simulink model "acados_test_old"  (R2017b)
settings: Solver=FixedStepDiscrete  StartTime=0.0  StopTime=200  FixedStep=1  RelTol=1e-3
PostLoadFcn:
  | , if any(exist('dsrtsu_mdlpostloadfcn', 'file') == [2, 3, 6]), try dsrtsu_mdlpostloadfcn('Execute', bdroot); catch fprintf('Error in PostLoadFcn (dsrtsu_mdlpostloadfcn) for model "%s":\n %s\n', bdroot, lasterr); end, end,
Description:
  | Standard RTI1401 template.
  | Supported MATLAB version:  R2017b.
settings Model: Tag=RTI1401  DSRTSU_INTERNAL_RTI_VER=520  DSRTSU_INTERNAL_RTI_TYPE=rti1401  RTICANMMDATA=struct('GeneralSetupData',struct('modelroot','D:\dSpace_Acados_Test','generalsettings',struct('filesettings',struct('destfolder',struct('Name','RTICANMM_FILES','Check',1),'buildfolder',struct('Name','.','Check',1),'AbsDestfolder',struct('Name','D:\dSpace_Acados_Test\RTICANMM_FILES'),'AbsBuildfolder',struct('Name','D:\dSpace_Acados_Test'))),'options',struct('addpaths',1,'rmpaths',1,'addtrcexclusion',logical(1),'cannavigator',struct('checkmonitoring',0),'show_usrtrc',0,'use_usrtrc',0),'advanced',struct('options',ones(1,100)),'MPSetup',{{}},'RTI',struct('Type','RTI1401','Ver','7.10','Date','02-May-2018'),'modelname','acados_test','block','acados_test'))  DSRTSU_INTERNAL_RTIFPGA=110  Creator=fleqscar  LastModifiedBy=fleqscar
settings SolverCC: AlgebraicLoopSolver=LineSearch
settings OptimizationCC: BlockReduction=off  OptimizeBlockIOStorage=off  BufferReuse=off  GlobalBufferReuse=off  ExpressionFolding=off  LocalBlockOutputs=off
settings HardwareCC: ProdBitPerPointer=32  ProdBitPerSizeT=32  ProdBitPerPtrDiffT=32  ProdLargestAtomicInteger=Integer  ProdEndianess=BigEndian  ProdWordSize=32  ProdHWDeviceType=Custom Processor->Custom  TargetIntDivRoundTo=Zero  TargetEndianess=BigEndian  TargetHWDeviceType=Custom Processor->Custom
settings SFSimCC: MATLABDynamicMemAlloc=off
settings RTWCC: SystemTargetFile=rti1401.tlc  MakeCommand=make_rti  TemplateMakefile=rti1401.tmf  Description=dSPACE DS1401 Hardware Platform
settings CodeAppCC: StateflowObjectComments=on
settings STFCustomTargetCC: ParMdlRefBuildCompliant=on  GRTInterface=off  SystemTargetFile=rti1401.tlc
settings GRTTargetCC: TargetLangStandard=C89/C90 (ANSI)  CompOptLevelCompliant=off  ConcurrentExecutionCompliant=off  CombineOutputUpdateFcns=off  MatFileLogging=off  CPPClassGenCompliant=off  UseToolchainInfoCompliant=off
settings ConfigComp: CovMetricSettings=dswe

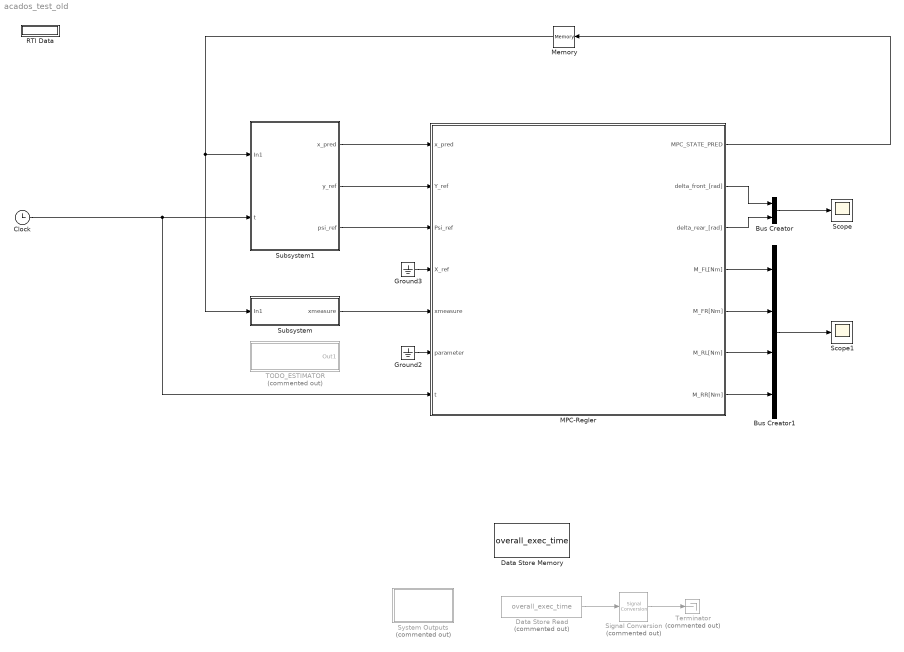
== system acados_test_old ==
  Bus Creator : BusCreator  Inputs=2
  Bus Creator1 : BusCreator  Inputs=4
  Clock : Clock
  Data Store Memory : DataStoreMemory  DataStoreName=overall_exec_time  ReadBeforeWriteMsg=warning  WriteAfterWriteMsg=warning  WriteAfterReadMsg=warning  ShowAdditionalParam=off
  Data Store Read : DataStoreRead  Commented=on  DataStoreName=overall_exec_time
  Ground2 : Ground
  Ground3 : Ground
  MPC-Regler : Subsystem  TreatAsAtomicUnit=on
  Memory : Memory
  RTI Data : Subsystem  Tag=struct('RTIDataServer',struct('RTIDataServerVs','2','RTIModelDescription','struct(''main'',''acados_test'',''sub'','''',''isMp'',0)'))  LoadFcn="if exist('rtidc'), try,  rtidc('DataHostBlockClbLoad', gcbh); catch, disp(['Warning: ''LoadFcn'' for RTI Data block failed: ' lasterr]); end, end,"  mask(RTI_DATA_HOST){}
      mask help:
      | RTI Data Block.
      | This block is used by RTI to store internal model-dependent data.
      | Please keep this block on the root level of the model. Deleting this block will result in data loss.
      |
      | NEVER DELETE OR COPY THIS BLOCK!
      settings: CopyFcn="if exist('rtidc'), try,  rtidc('DataHostBlockClbCopy', gcbh); catch, disp(['Warning: ''CopyFcn'' for RTI Data block failed: ' lasterr]); end, end,"  DeleteFcn="if exist('rtidc'), try,  rtidc('DataHostBlockClbDelete', gcbh); catch, disp(['Warning: ''DeleteFcn'' for RTI Data block failed: ' lasterr]); end, end,"  ModelCloseFcn="if exist('rtidc'), try,  rtidc('DataHostBlockClbModelClose', gcbh); catch, disp(['Warning: ''ModelCloseFcn'' for RTI Data block failed: ' lasterr]); end, end,"  PreSaveFcn="if exist('rtidc'), try,  rtidc('DataHostBlockClbPreSave', gcbh); catch, disp(['Warning: ''PreSaveFcn'' for RTI Data block failed: ' lasterr]); end, end,"  PostSaveFcn="if exist('rtidc'), try,  rtidc('DataHostBlockClbPostSave', gcbh); catch, disp(['Warning: ''PostSaveFcn'' for RTI Data block failed: ' lasterr]); end, end,"  NameChangeFcn="if exist('rtidc'), try,  rtidc('DataHostBlockClbNameChange', gcbh); catch, disp(['Warning: ''NameChangeFcn'' for RTI Data block failed: ' lasterr]); end, end,"
      mask Help:
      | RTI Data Block.
      | This block is used by RTI to store internal model-dependent data.
      | Please keep this block on the root level of the model. Deleting this block will result in data loss.
      | 
      | NEVER DELETE OR COPY THIS BLOCK!
      mask Display:
      | text(0.5, 0.5, 'RTI Data', 'HorizontalAlignment', 'center');
      | plot([1 0]);
  Scope : Scope
  Scope1 : Scope
  Signal Conversion : SignalConversion  Commented=on  OverrideOpt=off
  Subsystem : Subsystem  TreatAsAtomicUnit=on
  Subsystem1 : Subsystem  InitFcn=x_pred = 0:0.1:4.9;
  System Outputs : Subsystem  Commented=on  mask(System Outputs){ShowInLibBrowser=0}
      mask prompts: ShowInLibBrowser "Simulink:masks:CustCodeMaskParam1_MP"
      settings: CopyFcn=cccopyfcn(gcb)  OpenFcn=ccopenfcn('System Outputs Function')
      mask Help: eval('feval(''rtwprivate'',''rtwhelpview'',''rtw_sys_outputs_block'')');
      mask Display: disp('System\nOutputs');
  TODO_ESTIMATOR : Subsystem  Commented=on  TreatAsAtomicUnit=on
  Terminator : Terminator  Commented=on
  wires:
  Ground2/1 -> MPC-Regler/6(parameter)
  Signal Conversion/1 -> Terminator/1
  Data Store Read/1 -> Signal Conversion/1
  Subsystem1/2(y_ref) -> MPC-Regler/2(Y_ref)
  Subsystem1/1("x_pred ") -> MPC-Regler/1(x_pred)
  Subsystem/1(xmeasure) -> MPC-Regler/5(xmeasure)
  Ground3/1 -> MPC-Regler/4(X_ref)
  Clock/1 -> MPC-Regler/7(t), Subsystem1/2(t)
  Subsystem1/3(psi_ref) -> MPC-Regler/3(Psi_ref)
  Memory/1 -> Subsystem/1(In1), Subsystem1/1(In1)
  MPC-Regler/1(MPC_STATE_PRED) -> Memory/1
  MPC-Regler/2(" delta_front_[rad]") -> Bus Creator/1
  MPC-Regler/3(" delta_rear_[rad]") -> Bus Creator/2
  Bus Creator/1 -> Scope/1
  MPC-Regler/4(M_FL[Nm]) -> Bus Creator1/1
  MPC-Regler/5(M_FR[Nm]) -> Bus Creator1/2
  MPC-Regler/6(M_RL[Nm]) -> Bus Creator1/3
  MPC-Regler/7(M_RR[Nm]) -> Bus Creator1/4
  Bus Creator1/1 -> Scope1/1

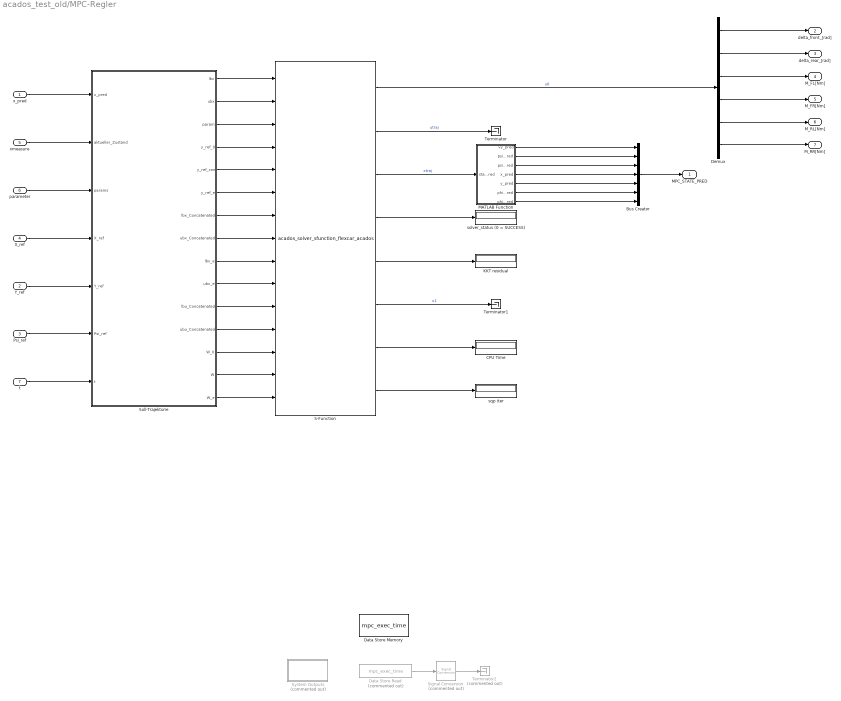
== system acados_test_old/MPC-Regler ==
  x_pred : Inport
  Y_ref : Inport  Port=2
  Psi_ref : Inport  Port=3
  X_ref : Inport  Port=4
  xmeasure : Inport  Port=5
  parameter : Inport  Port=6
  t : Inport  Port=7
  Bus Creator : BusCreator  Inputs=7
  CPU Time : Display
  Data Store Memory : DataStoreMemory  DataStoreName=mpc_exec_time  ReadBeforeWriteMsg=warning  WriteAfterWriteMsg=warning  WriteAfterReadMsg=warning  ShowAdditionalParam=off
  Data Store Read : DataStoreRead  Commented=on  DataStoreName=mpc_exec_time
  Demux : Demux  Outputs=6
  KKT residual : Display
  MATLAB Function : MATLAB Function  TreatAsAtomicUnit=on
  S-Function : S-Function  FunctionName=acados_solver_sfunction_flexcar_acados  SFunctionDeploymentMode=off  EnableBusSupport=off
  Signal Conversion : SignalConversion  Commented=on  OverrideOpt=off
  Soll-Trajektorie : Subsystem  TreatAsAtomicUnit=on
  System Outputs : Subsystem  Commented=on  mask(System Outputs){ShowInLibBrowser=0}
      mask prompts: ShowInLibBrowser "Simulink:masks:CustCodeMaskParam1_MP"
      settings: CopyFcn=cccopyfcn(gcb)  OpenFcn=ccopenfcn('System Outputs Function')
      mask Help: eval('feval(''rtwprivate'',''rtwhelpview'',''rtw_sys_outputs_block'')');
      mask Display: disp('System\nOutputs');
  Terminator : Terminator
  Terminator1 : Terminator
  Terminator2 : Terminator  Commented=on
  solver_status (0 = SUCCESS) : Display
  sqp iter : Display
  MPC_STATE_PRED : Outport
  " delta_front_[rad]" : Outport  Port=2
  " delta_rear_[rad]" : Outport  Port=3
  M_FL[Nm] : Outport  Port=4
  M_FR[Nm] : Outport  Port=5
  M_RL[Nm] : Outport  Port=6
  M_RR[Nm] : Outport  Port=7
  wires:
  Soll-Trajektorie/10(ubx_e) -> S-Function/10
  Soll-Trajektorie/9(lbx_e) -> S-Function/9
  Soll-Trajektorie/4(y_ref_0) -> S-Function/4
  Soll-Trajektorie/15(W_e) -> S-Function/15
  Soll-Trajektorie/6(y_ref_e) -> S-Function/6
  Soll-Trajektorie/2(ubx) -> S-Function/2
  Soll-Trajektorie/7(lbx_Concatenated) -> S-Function/7
  Soll-Trajektorie/12(ubu_Concatenated) -> S-Function/12
  Soll-Trajektorie/3(param) -> S-Function/3
  Soll-Trajektorie/8(ubx_Concatenated) -> S-Function/8
  Soll-Trajektorie/13(W_0) -> S-Function/13
  Soll-Trajektorie/1(lbx) -> S-Function/1
  Soll-Trajektorie/11(lbu_Concatenated) -> S-Function/11
  Soll-Trajektorie/5(y_ref_con) -> S-Function/5
  Soll-Trajektorie/14(W) -> S-Function/14
  x_pred/1 -> Soll-Trajektorie/1(x_pred)
  parameter/1 -> Soll-Trajektorie/3(params)
  xmeasure/1 -> Soll-Trajektorie/2(aktueller_Zustand)
  X_ref/1 -> Soll-Trajektorie/4("X_ref ")
  Y_ref/1 -> Soll-Trajektorie/5(Y_ref)
  t/1 -> Soll-Trajektorie/7(t)
  Psi_ref/1 -> Soll-Trajektorie/6(Psi_ref)
  S-Function/7 -> CPU Time/1
  Demux/2 -> " delta_rear_[rad]"/1
  Demux/1 -> " delta_front_[rad]"/1
  Demux/4 -> M_FR[Nm]/1
  S-Function/2 -> Terminator/1  "utraj"
  MATLAB Function/7(phi_pred) -> Bus Creator/7
  Bus Creator/1 -> MPC_STATE_PRED/1
  S-Function/4 -> solver_status (0 = SUCCESS)/1
  MATLAB Function/1(vy_pred) -> Bus Creator/1
  S-Function/8 -> sqp iter/1
  S-Function/1 -> Demux/1  "u0"
  S-Function/6 -> Terminator1/1  "x1"
  MATLAB Function/4(x_pred) -> Bus Creator/4
  MATLAB Function/6(phidot_pred) -> Bus Creator/6
  MATLAB Function/2(psidot_pred) -> Bus Creator/2
  S-Function/3 -> MATLAB Function/1(state_pred)  "xtraj"
  Demux/3 -> M_FL[Nm]/1
  MATLAB Function/3(psi_pred) -> Bus Creator/3
  Demux/6 -> M_RR[Nm]/1
  Demux/5 -> M_RL[Nm]/1
  S-Function/5 -> KKT residual/1
  MATLAB Function/5(y_pred) -> Bus Creator/5
  Signal Conversion/1 -> Terminator2/1
  Data Store Read/1 -> Signal Conversion/1

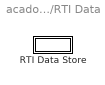
== system acados_test_old/RTI Data ==
  RTI Data Store : Subsystem  Tag="struct('private',struct('version',struct('dsVer',uint32(2),'dsVerCreation',uint32(2),'RTI',struct('ver','7.10','type','RTI1401')),'access',struct('type','Model','isPerm',1,'created',['24-Apr-2021 13:44:56'],'modified',['14-May-2021 12:55:04'],'location','')),'public',struct('main',struct('data',[]),'sub',struct('name',{{'acados_test'}},'data',{{struct('TH',struct('thTaskInfo',struct('taskType',{'TIMER','HWINT','TMRINT','SWINT','GLINT'},'tasksNumOf',{1,0,0,0,0},'srcIds',{{'TIMERA'},{},{},{},{}},'taskNames',{{['Timer Task 1']},{},{},{},{}})),'th_tc',struct('dataType','TASK','taskGroupId','','taskGroupList',{{}},'taskSchedulingPolicy','FCFS','taskType','TIMER','blkh',-1,'srcId','TIMERA','srcSgnName',['Timer A interrupt'],'srcCpuName','','taskName',['Timer Task 1  [1] s'],'taskNameDisplayExt','','smplTime',1,'smplTimeOffs',0,'hasFixedPriority',0,'priority',1,'hasFixedOvc',0,'ovcType',1,'ovcMax',1),'tc_th',struct('dataType','TASK','taskGroupId','','taskGroupList',{{}},'taskSchedulingPolicy','FCFS','taskType','TIMER','blkh',-1,'srcId','TIMERA','srcSgnName',['Timer A interrupt'],'srcCpuName','','taskName',['Timer Task 1  [1] s'],'taskNameDisplayExt','','smplTime',1,'smplTimeOffs',0,'hasFixedPriority',0,'priority',1,'hasFixedOvc',0,'ovcType',1,'ovcMax',1))}})))"  mask(RTI_DATA_STORE){}
      mask help:
      | RTI Data Store Block. This block is used by RTI to store internal model dependent data. Deleting this block will result in data loss.
      |
      | NEVER DELETE, COPY, OR MODIFY THIS BLOCK!
      mask Help:
      | RTI Data Store Block. This block is used by RTI to store internal model dependent data. Deleting this block will result in data loss.
      | 
      | NEVER DELETE, COPY, OR MODIFY THIS BLOCK!
      mask Display: text(0.5, 0.5, ' ', 'HorizontalAlignment', 'center');

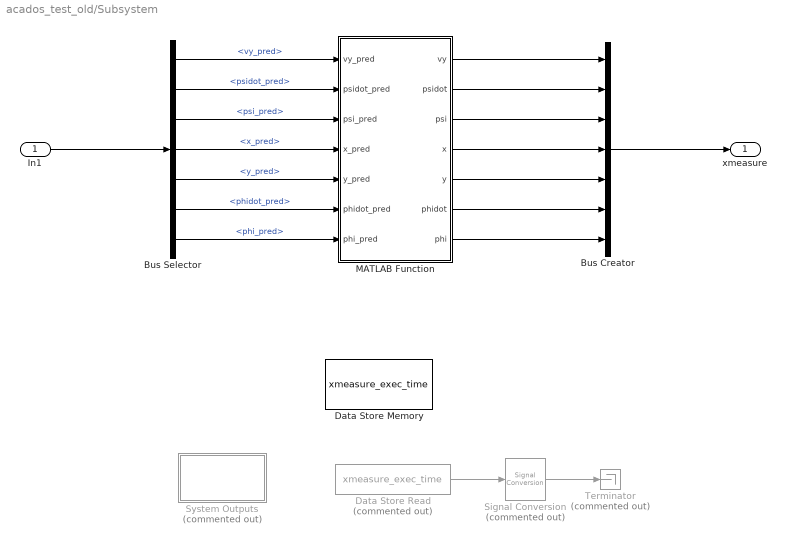
== system acados_test_old/Subsystem ==
  In1 : Inport
  Bus Creator : BusCreator  Inputs=7
  Bus Selector : BusSelector  OutputSignals=vy_pred,psidot_pred,psi_pred,x_pred,y_pred,phidot_pred,phi_pred
  Data Store Memory : DataStoreMemory  DataStoreName=xmeasure_exec_time  ReadBeforeWriteMsg=warning  WriteAfterWriteMsg=warning  WriteAfterReadMsg=warning  ShowAdditionalParam=off
  Data Store Read : DataStoreRead  Commented=on  DataStoreName=xmeasure_exec_time
  MATLAB Function : MATLAB Function  TreatAsAtomicUnit=on
  Signal Conversion : SignalConversion  Commented=on  OverrideOpt=off
  System Outputs : Subsystem  Commented=on  mask(System Outputs){ShowInLibBrowser=0}
      mask prompts: ShowInLibBrowser "Simulink:masks:CustCodeMaskParam1_MP"
      settings: CopyFcn=cccopyfcn(gcb)  OpenFcn=ccopenfcn('System Outputs Function')
      mask Help: eval('feval(''rtwprivate'',''rtwhelpview'',''rtw_sys_outputs_block'')');
      mask Display: disp('System\nOutputs');
  Terminator : Terminator  Commented=on
  xmeasure : Outport
  wires:
  In1/1 -> Bus Selector/1
  Bus Selector/1 -> MATLAB Function/1(vy_pred)  "<vy_pred>"
  Bus Selector/2 -> MATLAB Function/2(psidot_pred)  "<psidot_pred>"
  Bus Selector/3 -> MATLAB Function/3(psi_pred)  "<psi_pred>"
  Bus Selector/4 -> MATLAB Function/4(x_pred)  "<x_pred>"
  Bus Selector/5 -> MATLAB Function/5(y_pred)  "<y_pred>"
  Bus Selector/6 -> MATLAB Function/6(phidot_pred)  "<phidot_pred>"
  Bus Selector/7 -> MATLAB Function/7(phi_pred)  "<phi_pred>"
  MATLAB Function/1(vy) -> Bus Creator/1
  MATLAB Function/2(psidot) -> Bus Creator/2
  MATLAB Function/3(psi) -> Bus Creator/3
  MATLAB Function/4(x) -> Bus Creator/4
  MATLAB Function/5(y) -> Bus Creator/5
  MATLAB Function/6(phidot) -> Bus Creator/6
  MATLAB Function/7(phi) -> Bus Creator/7
  Bus Creator/1 -> xmeasure/1
  Signal Conversion/1 -> Terminator/1
  Data Store Read/1 -> Signal Conversion/1

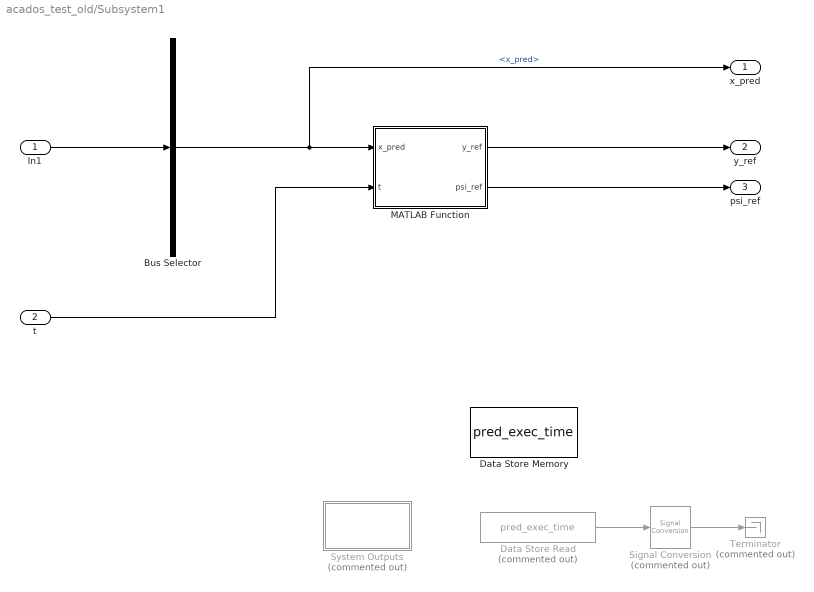
== system acados_test_old/Subsystem1 ==
  In1 : Inport
  t : Inport  Port=2
  Bus Selector : BusSelector  OutputSignals=x_pred
  Data Store Memory : DataStoreMemory  DataStoreName=pred_exec_time  ReadBeforeWriteMsg=warning  WriteAfterWriteMsg=warning  WriteAfterReadMsg=warning  ShowAdditionalParam=off
  Data Store Read : DataStoreRead  Commented=on  DataStoreName=pred_exec_time
  MATLAB Function : MATLAB Function  TreatAsAtomicUnit=on
  Signal Conversion : SignalConversion  Commented=on  OverrideOpt=off
  System Outputs : Subsystem  Commented=on  mask(System Outputs){ShowInLibBrowser=0}
      mask prompts: ShowInLibBrowser "Simulink:masks:CustCodeMaskParam1_MP"
      settings: CopyFcn=cccopyfcn(gcb)  OpenFcn=ccopenfcn('System Outputs Function')
      mask Help: eval('feval(''rtwprivate'',''rtwhelpview'',''rtw_sys_outputs_block'')');
      mask Display: disp('System\nOutputs');
  Terminator : Terminator  Commented=on
  "x_pred " : Outport
  y_ref : Outport  Port=2
  psi_ref : Outport  Port=3
  wires:
  In1/1 -> Bus Selector/1
  Bus Selector/1 -> "x_pred "/1, MATLAB Function/1(x_pred)  "<x_pred>"
  MATLAB Function/1(y_ref) -> y_ref/1
  MATLAB Function/2(psi_ref) -> psi_ref/1
  t/1 -> MATLAB Function/2(t)
  Signal Conversion/1 -> Terminator/1
  Data Store Read/1 -> Signal Conversion/1

== system acados_test_old/System Outputs ==

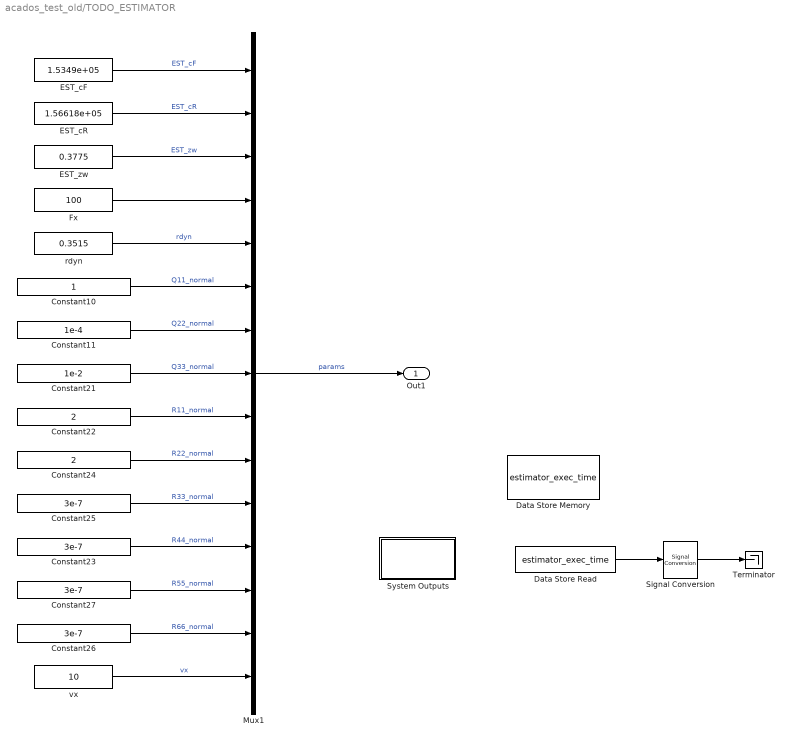
== system acados_test_old/TODO_ESTIMATOR ==
  Constant10 : Constant  SampleTime=-1
  Constant11 : Constant  Value=1e-4  SampleTime=-1
  Constant21 : Constant  Value=1e-2  SampleTime=-1
  Constant22 : Constant  Value=2  SampleTime=-1
  Constant{23,25..27} (4 alike) : Constant  Value=3e-7  SampleTime=-1
  Constant24 : Constant  Value=2  SampleTime=-1
  Data Store Memory : DataStoreMemory  DataStoreName=estimator_exec_time  ReadBeforeWriteMsg=warning  WriteAfterWriteMsg=warning  WriteAfterReadMsg=warning  ShowAdditionalParam=off
  Data Store Read : DataStoreRead  DataStoreName=estimator_exec_time
  EST_cF : Constant  Value=1.5349e+05  SampleTime=-1
  EST_cR : Constant  Value=1.56618e+05  SampleTime=-1
  EST_zw : Constant  Value=0.3775  SampleTime=-1
  Fx : Constant  Value=100  SampleTime=-1
  Mux1 : Mux  Inputs=15
  Signal Conversion : SignalConversion  OverrideOpt=off
  System Outputs : Subsystem  mask(System Outputs){ShowInLibBrowser=0}
      mask prompts: ShowInLibBrowser "Simulink:masks:CustCodeMaskParam1_MP"
      settings: CopyFcn=cccopyfcn(gcb)  OpenFcn=ccopenfcn('System Outputs Function')
      mask Help: eval('feval(''rtwprivate'',''rtwhelpview'',''rtw_sys_outputs_block'')');
      mask Display: disp('System\nOutputs');
  Terminator : Terminator
  rdyn : Constant  Value=0.3515  SampleTime=-1
  vx : Constant  Value=10  SampleTime=-1
  Out1 : Outport
  wires:
  Fx/1 -> Mux1/4
  Constant24/1 -> Mux1/10  "R22_normal"
  EST_cF/1 -> Mux1/1  "EST_cF"
  EST_cR/1 -> Mux1/2  "EST_cR"
  Constant21/1 -> Mux1/8  "Q33_normal"
  Constant26/1 -> Mux1/14  "R66_normal"
  Constant23/1 -> Mux1/12  "R44_normal"
  Constant22/1 -> Mux1/9  "R11_normal"
  EST_zw/1 -> Mux1/3  "EST_zw"
  Constant25/1 -> Mux1/11  "R33_normal"
  Mux1/1 -> Out1/1  "params"
  vx/1 -> Mux1/15  "vx"
  Constant10/1 -> Mux1/6  "Q11_normal"
  rdyn/1 -> Mux1/5  "rdyn"
  Constant11/1 -> Mux1/7  "Q22_normal"
  Constant27/1 -> Mux1/13  "R55_normal"
  Data Store Read/1 -> Signal Conversion/1
  Signal Conversion/1 -> Terminator/1

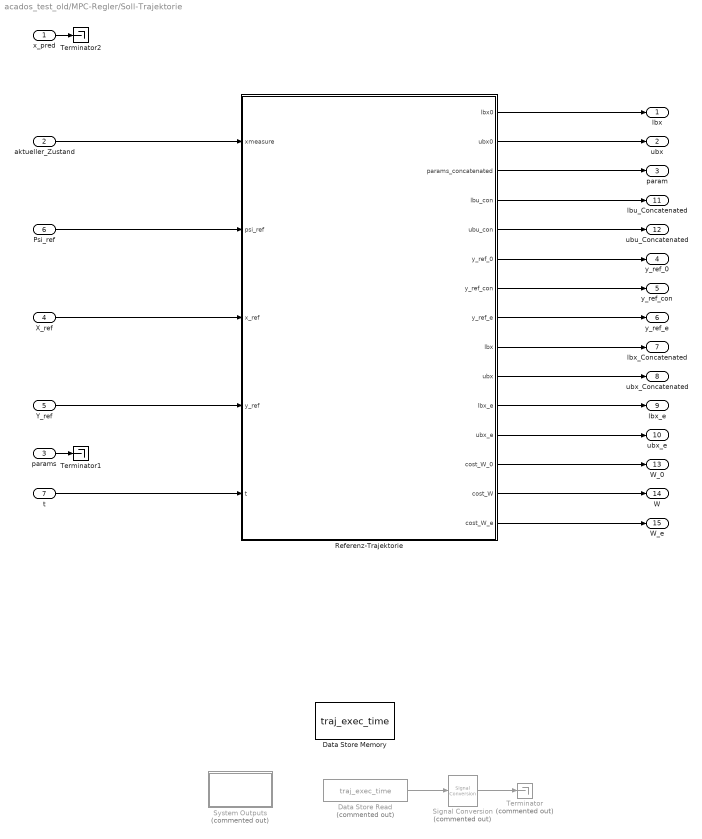
== system acados_test_old/MPC-Regler/Soll-Trajektorie ==
  x_pred : Inport
  aktueller_Zustand : Inport  Port=2
  params : Inport  Port=3
  "X_ref " : Inport  Port=4
  Y_ref : Inport  Port=5
  Psi_ref : Inport  Port=6
  t : Inport  Port=7
  Data Store Memory : DataStoreMemory  DataStoreName=traj_exec_time  ReadBeforeWriteMsg=warning  WriteAfterWriteMsg=warning  WriteAfterReadMsg=warning  ShowAdditionalParam=off
  Data Store Read : DataStoreRead  Commented=on  DataStoreName=traj_exec_time
  Referenz-Trajektorie : MATLAB Function  TreatAsAtomicUnit=on
  Signal Conversion : SignalConversion  Commented=on  OverrideOpt=off
  System Outputs : Subsystem  Commented=on  mask(System Outputs){ShowInLibBrowser=0}
      mask prompts: ShowInLibBrowser "Simulink:masks:CustCodeMaskParam1_MP"
      settings: CopyFcn=cccopyfcn(gcb)  OpenFcn=ccopenfcn('System Outputs Function')
      mask Help: eval('feval(''rtwprivate'',''rtwhelpview'',''rtw_sys_outputs_block'')');
      mask Display: disp('System\nOutputs');
  Terminator : Terminator  Commented=on
  Terminator1 : Terminator
  Terminator2 : Terminator
  lbx : Outport
  ubx : Outport  Port=2
  param : Outport  Port=3
  y_ref_0 : Outport  Port=4
  y_ref_con : Outport  Port=5
  y_ref_e : Outport  Port=6
  lbx_Concatenated : Outport  Port=7
  ubx_Concatenated : Outport  Port=8
  lbx_e : Outport  Port=9
  ubx_e : Outport  Port=10
  lbu_Concatenated : Outport  Port=11
  ubu_Concatenated : Outport  Port=12
  W_0 : Outport  Port=13
  W : Outport  Port=14
  W_e : Outport  Port=15
  wires:
  aktueller_Zustand/1 -> Referenz-Trajektorie/1(xmeasure)
  Referenz-Trajektorie/3(params_concatenated) -> param/1
  Psi_ref/1 -> Referenz-Trajektorie/2(psi_ref)
  "X_ref "/1 -> Referenz-Trajektorie/3(x_ref)
  Y_ref/1 -> Referenz-Trajektorie/4(y_ref)
  Referenz-Trajektorie/5(ubu_con) -> ubu_Concatenated/1
  Referenz-Trajektorie/4(lbu_con) -> lbu_Concatenated/1
  Referenz-Trajektorie/6(y_ref_0) -> y_ref_0/1
  Referenz-Trajektorie/7(y_ref_con) -> y_ref_con/1
  Referenz-Trajektorie/8(y_ref_e) -> y_ref_e/1
  Referenz-Trajektorie/15(cost_W_e) -> W_e/1
  Referenz-Trajektorie/14(cost_W) -> W/1
  Referenz-Trajektorie/13(cost_W_0) -> W_0/1
  Referenz-Trajektorie/9(lbx) -> lbx_Concatenated/1
  Referenz-Trajektorie/10(ubx) -> ubx_Concatenated/1
  Referenz-Trajektorie/11(lbx_e) -> lbx_e/1
  Referenz-Trajektorie/12(ubx_e) -> ubx_e/1
  t/1 -> Referenz-Trajektorie/5(t)
  Referenz-Trajektorie/1(lbx0) -> lbx/1
  Referenz-Trajektorie/2(ubx0) -> ubx/1
  Signal Conversion/1 -> Terminator/1
  Data Store Read/1 -> Signal Conversion/1
  params/1 -> Terminator1/1
  x_pred/1 -> Terminator2/1

== system acados_test_old/MPC-Regler/System Outputs ==

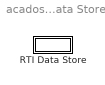
== system acados_test_old/RTI Data/RTI Data Store ==
  RTI Data Store : Subsystem  mask(RTI_DATA_STORE){}
      mask help:
      | RTI Data Store Block. This block is used by RTI to store internal model dependent data. Deleting this block will result in data loss.
      |
      | NEVER DELETE, COPY, OR MODIFY THIS BLOCK!
      mask Help:
      | RTI Data Store Block. This block is used by RTI to store internal model dependent data. Deleting this block will result in data loss.
      | 
      | NEVER DELETE, COPY, OR MODIFY THIS BLOCK!
      mask Display: text(0.5, 0.5, ' ', 'HorizontalAlignment', 'center');

== system acados_test_old/Subsystem/System Outputs ==

== system acados_test_old/Subsystem1/System Outputs ==

== system acados_test_old/TODO_ESTIMATOR/System Outputs ==

== system acados_test_old/MPC-Regler/Soll-Trajektorie/System Outputs ==

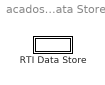
== system acados_test_old/RTI Data/RTI Data Store/RTI Data Store ==
  RTI Data Store : Subsystem  mask(RTI_DATA_STORE){}
      mask help:
      | RTI Data Store Block. This block is used by RTI to store internal model dependent data. Deleting this block will result in data loss.
      |
      | NEVER DELETE, COPY, OR MODIFY THIS BLOCK!
      mask Help:
      | RTI Data Store Block. This block is used by RTI to store internal model dependent data. Deleting this block will result in data loss.
      | 
      | NEVER DELETE, COPY, OR MODIFY THIS BLOCK!
      mask Display: text(0.5, 0.5, ' ', 'HorizontalAlignment', 'center');

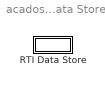
== system acados_test_old/RTI Data/RTI Data Store/RTI Data Store/RTI Data Store ==
  RTI Data Store : Subsystem  mask(RTI_DATA_STORE){}
      mask help:
      | RTI Data Store Block. This block is used by RTI to store internal model dependent data. Deleting this block will result in data loss.
      |
      | NEVER DELETE, COPY, OR MODIFY THIS BLOCK!
      mask Help:
      | RTI Data Store Block. This block is used by RTI to store internal model dependent data. Deleting this block will result in data loss.
      | 
      | NEVER DELETE, COPY, OR MODIFY THIS BLOCK!
      mask Display: text(0.5, 0.5, ' ', 'HorizontalAlignment', 'center');

== system acados_test_old/RTI Data/RTI Data Store/RTI Data Store/RTI Data Store/RTI Data Store ==

== matlab function acados_test_old/MPC-Regler/MATLAB Function ==
  data: state_pred input size=[147, 1]; vy_pred output; psidot_pred output; psi_pred output; x_pred output; y_pred output; phidot_pred output; phi_pred output
function [vy_pred, psidot_pred, psi_pred, x_pred, y_pred, phidot_pred, phi_pred] = fcn(state_pred)

N = 20;
st_pred = zeros(7, N+1);
st_pred = reshape(state_pred, 7, N+1);

vy_pred = st_pred(1, 1:N);
psidot_pred = st_pred(2, 1:N);
psi_pred = st_pred(3, 1:N);
x_pred = st_pred(4, 1:N);
y_pred = st_pred(5, 1:N);
phidot_pred = st_pred(6, 1:N);
phi_pred = st_pred(7, 1:N);

end

== matlab function acados_test_old/MPC-Regler/Soll-Trajektorie/Referenz-Trajektorie ==
  data: lbx0 output; ubx0 output; xmeasure input; psi_ref input; x_ref input; y_ref input; params_concatenated output size=[1, 63]; lbu_con output; ubu_con output; y_ref_0 output; y_ref_con output; y_ref_e output; lbx output size=[1, 38]; ubx output size=[1, 38]; lbx_e output size=[1, 2]; ubx_e output size=[1, 2]; cost_W_0 output size=[1, 196]; cost_W output size=[1, 196]; cost_W_e output size=[1, 49]; t input
function [lbx0, ubx0, params_concatenated, lbu_con, ubu_con, y_ref_0, y_ref_con, y_ref_e, ...
          lbx, ubx, lbx_e, ubx_e, cost_W_0, cost_W, cost_W_e]  = fcn(xmeasure, psi_ref, x_ref, y_ref, t)

lbx0 = xmeasure; 
ubx0 = xmeasure; 
      
lbu = [-deg2rad(23),-deg2rad(23), -50, -50, -50, -50]';
param = [1.5349e+05, 1.56618e+05, 0.3775, 100, 0.315, 1, 1e-4, 1e-2, 2, 2, 3e-7, 3e-7, 3e-7, 3e-7, 10];
nx = 7; 
nu = 6;
n_M = 1; 
nz = 0;
N = 20;

Fx_ref = param(4);
rdyn = param(5);

% if t < 0.01
%     vx = 3; %for t=0, vx = 0 and therefore dynamics -> inf
% else
%     vx = param(15);
% end

vx = param(15);

Q_11 = param(6); 
Q_22 = param(7); 
Q_33 = param(8); 
R_11 = param(9); 
R_22 = param(10); 
R_33 = param(11); 
R_44 = param(12); 
R_55 = param(13); 
R_66 = param(14); 


% param0 = [x_ref'; y_ref'; psi_ref'; Fx_ref; rdyn];
param0 = [Fx_ref; rdyn; vx];
params_concatenated = repmat(param0, N+1, 1)';

lbu_con = repmat(lbu, N, 1);
ubu_con = -lbu_con;


%% Ref for Optimization Variable Y = [X; U]
y_ref_0 = zeros(nx+nu+n_M, 1);
y_ref_0(3) = psi_ref(1);
y_ref_0(5) = y_ref(1);
y_ref_0(end) = Fx_ref;

y_ref_mat = zeros(nx+nu+n_M, N-1);
y_ref_mat(3, :) = psi_ref(2:end);
y_ref_mat(5, :) = y_ref(2:end);
y_ref_mat(end, :) = Fx_ref * ones(1, N-1)';
y_ref_con = reshape(y_ref_mat, (nx+nu+n_M)*(N-1), 1);

y_ref_e = zeros(nx, 1);
y_ref_e(3) = psi_ref(end);
y_ref_e(5) = y_ref(end);

Y_ref_lb = zeros(2, N-1);
Y_ref_ub = zeros(2, N-1);
Y_ref_lb(1, :) = y_ref_mat(3, :) - deg2rad(30); % -10deg 
Y_ref_lb(2, :) = y_ref_mat(5, :) - 1;         % -0.1m
Y_ref_ub(1, :) = y_ref_mat(3, :) + deg2rad(30); % +10deg 
Y_ref_ub(2, :) = y_ref_mat(5, :) + 1;         % +0.1m

% Reshape in column-major form (thats what reshape() does!)
lbx = reshape(Y_ref_lb, 1, 2*(N-1));
ubx = reshape(Y_ref_ub, 1, 2*(N-1));
lbx_e = [y_ref_e(3), y_ref_e(5)];
ubx_e = [y_ref_e(3), y_ref_e(5)];

%% WEIGHTING MATRICES
% W_x = diag([0; 0; p(3); 0; p(4); 0; 0]);
% W_u = diag(p(6:11));
% W_Mx = p(5);

COST_W_0 = zeros(nx+nu+n_M, nx+nu+n_M);
COST_W_e = zeros(nx, nx);

COST_W_0(3, 3) = Q_11;
COST_W_0(5, 5) = Q_22;
COST_W_0(8:13, 8:13) = diag([R_11, R_22, R_33, R_44, R_55, R_66]);
COST_W_0(14, 14) = Q_33;

COST_W_e = 10*COST_W_0(1:nx, 1:nx);

% Reshape in column-major form (thats what reshape() does!)
cost_W_0 = reshape(COST_W_0, 1, (nx+nu+n_M)*(nx+nu+n_M));
cost_W = cost_W_0;
cost_W_e = reshape(COST_W_e, 1, nx*nx);

== matlab function acados_test_old/Subsystem/MATLAB Function ==
  data: vy output; psidot output; psi output; x output; vy_pred input; y output; psidot_pred input; psi_pred input; x_pred input; y_pred input; phidot_pred input; phi_pred input; phidot output; phi output
function [vy, psidot, psi, x, y, phidot, phi] = fcn(vy_pred, psidot_pred, psi_pred, x_pred, y_pred, phidot_pred, phi_pred)

vy = vy_pred(2);
psidot = psidot_pred(2);
psi = psi_pred(2);
x = x_pred(2);
y = y_pred(2);
phidot = phidot_pred(2);
phi = phi_pred(2);



end

== matlab function acados_test_old/Subsystem1/MATLAB Function ==
  data: x_pred input; y_ref output; psi_ref output; t input
function [y_ref, psi_ref] = fcn(x_pred, t)

% if t < 0.025
%     x_pred = 0:0.1:4.9;
% end
[x_ref, x_upper_bound, x_lower_bound, Y_ref, Psi_ref] = get_referance();
% Y_ref = @(x) sin(0.1*x);
% Psi_ref = @(x) 0.1*cos(0.1*x);

y_ref = Y_ref(x_pred);
psi_ref = Psi_ref(x_pred);


end
function [x_ref, x_upper_bound, x_lower_bound, Y_ref, Psi_ref] = get_referance()
shape = 2.4;
d_x1 = 25;
d_x2 = 21.95;
d_y1 = 4.05; 
d_y2 = 5.7; 
Xs1 = 27.19; 
Xs2 = 56.46;

Psi_ref = @(X) atan(d_y1 * (1./cosh(shape/d_x1 * (X - Xs1) - shape/2)).^2 ...
            * (1.2/d_x1) - d_y2 * (1./cosh(shape/d_x2 * (X - Xs2) - shape/2)).^2 ...
            * (1.2/d_x2));
Psi_upper = @(X) atan(d_y1 * (1./cosh(shape/d_x1 * (X - Xs1) - shape/2)).^2 ...
            * (1.2/d_x1) - d_y2 * (1./cosh(shape/d_x2 * (X - Xs2) - shape/2)).^2 ...
            * (1.2/d_x2)) + deg2rad(30);    %max. = +5 deg. deviation from Psi_ref
Psi_lower = @(X) atan(d_y1 * (1./cosh(shape/d_x1 * (X - Xs1) - shape/2)).^2 ...
            * (1.2/d_x1) - d_y2 * (1./cosh(shape/d_x2 * (X - Xs2) - shape/2)).^2 ...
            * (1.2/d_x2)) - deg2rad(30);    %min. = -5 deg. deviation from Psi_ref
        
                
Y_ref = @(X) d_y1/2 * (1+tanh(shape/d_x1 * (X - Xs1) - shape/2)) ...
            - d_y2/2 * (1+tanh(shape/d_x2 * (X - Xs2) - shape/2));
Y_upper = @(X) d_y1/2 * (1+tanh(shape/d_x1 * (X - Xs1) - shape/2)) ...
            - d_y2/2 * (1+tanh(shape/d_x2 * (X - Xs2) - shape/2)) + 0.2; %max. =  +0.1m deviation from Y_ref       
Y_lower = @(X) d_y1/2 * (1+tanh(shape/d_x1 * (X - Xs1) - shape/2)) ...
            - d_y2/2 * (1+tanh(shape/d_x2 * (X - Xs2) - shape/2)) - 0.2; %min. =  -0.1m deviation from Y_ref       

     
x_ref = {Y_ref; Psi_ref};   

x_upper_bound = {Y_upper; Psi_upper};

x_lower_bound = {Y_lower; Psi_lower};   

end
